simulink model "time"  (R2020b)
settings: Solver=VariableStepAuto  StartTime=0.0  StopTime=10.0  RelTol=1e-3
libraries: dspnetwork x2
settings Model: Creator=xinbo  LastModifiedBy=xinbo

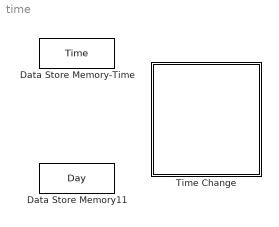
== system time ==
  Data Store Memory11 : DataStoreMemory  DataStoreName=Day  ReadBeforeWriteMsg=warning  WriteAfterWriteMsg=warning  WriteAfterReadMsg=warning  ShowAdditionalParam=off  OutDataTypeStr=double
  Data Store Memory-Time : DataStoreMemory  DataStoreName=Time  ReadBeforeWriteMsg=warning  WriteAfterWriteMsg=warning  WriteAfterReadMsg=warning  ShowAdditionalParam=off  OutDataTypeStr=double
  Time Change : Subsystem
      mask Display: image('/Users/xinbo/E/paper3/program_clean/digital_twin/images/time.png'); % Use "Edit Image" on toolstrip to change.

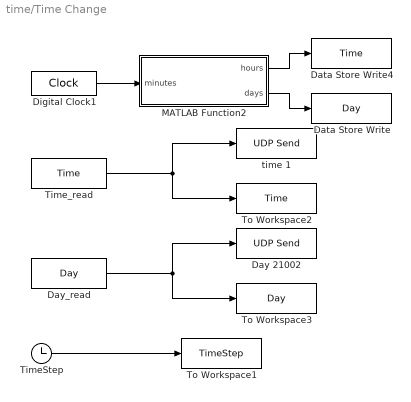
== system time/Time Change ==
  Data Store Write : DataStoreWrite  DataStoreName=Day
  Data Store Write4 : DataStoreWrite  DataStoreName=Time  SampleTime=1
  Day 21002 : dspnetwork/UDP Send  remoteURL='127.0.0.1'  remotePort=21002  localURL='0.0.0.0'  localPortSource=Automatically determine  localPort=-1  sendBufferSize=8192  sampletime=-1  blockPlatform=[]  separateLengthPort=0
  Day_read : DataStoreRead  DataStoreName=Day
  Digital Clock1 : DigitalClock
  MATLAB Function2 : MATLAB Function  TreatAsAtomicUnit=on
  TimeStep : Clock
  Time_read : DataStoreRead  DataStoreName=Time  SampleTime=1
  To Workspace1 : ToWorkspace  VariableName=TimeStep  SampleTime=-1
      settings: Save2DSignal=2-D array (concatenate along first dimension)
  To Workspace2 : ToWorkspace  VariableName=Time  SampleTime=-1
  To Workspace3 : ToWorkspace  VariableName=Day  SampleTime=-1
  time 1 : dspnetwork/UDP Send  remoteURL='127.0.0.1'  remotePort=21001  localURL='0.0.0.0'  localPortSource=Automatically determine  localPort=-1  sendBufferSize=8192  sampletime=-1  blockPlatform=[]  separateLengthPort=0
  wires:
  MATLAB Function2/2(days) -> Data Store Write/1
  MATLAB Function2/1(hours) -> Data Store Write4/1
  Time_read/1 -> time 1/1, To Workspace2/1
  Day_read/1 -> Day 21002/1, To Workspace3/1
  Digital Clock1/1 -> MATLAB Function2/1(minutes)
  TimeStep/1 -> To Workspace1/1

== matlab function time/Time Change/MATLAB Function2 ==
  data: minutes input; hours output; days output
function [hours, days]= calTime(minutes)

hours = minutes/60;
days = 0;

while(hours > 24)
    hours = hours - 24;
    days = days + 1;
end
